simulink model "Ejercicio_1_DB_Inicial"  (R2023a)
settings: Solver=VariableStepAuto  StartTime=0.0  StopTime=150  RelTol=1e-6
values from neighbouring files (symbols this model uses):
  A = 10    [Ejercicio_1.m]    (also in Ejercicio_2y3.m)
  A1 = 1e-2    (= 0.01)    [Ejercicio_1.m]    (also in Ejercicio_2y3.m)
  A2 = 1    [Ejercicio_1.m]    (also in Ejercicio_2y3.m)
  bT = bm + (R*A1)^2*Rh + (R*A1/A2)^2*bp    (= 6.227045)    [Ejercicio_1.m]    (also in Ejercicio_2y3.m)
  JT = Jm + Jr + R^2*mp + (R*A1/A2)^2*m    (= 4.5108)    [Ejercicio_1.m]    (also in Ejercicio_2y3.m)
  Kb = 1    [Ejercicio_1.m]    (also in Ejercicio_2y3.m)
  kP = 5    [Ejercicio_1.m]    (also in Ejercicio_2y3.m)
  Kt = 1    [Ejercicio_1.m]    (also in Ejercicio_2y3.m)
  kT = (R*A1)^2/Ch + (R*A1/A2)^2*km    (= 0.26829)    [Ejercicio_1.m]    (also in Ejercicio_2y3.m)
  La = 100e-3    (= 0.1)    [Ejercicio_1.m]    (also in Ejercicio_2y3.m)
  R = 0.3    [Ejercicio_1.m]    (also in Ejercicio_2y3.m)
  Ra = 2.1    [Ejercicio_1.m]    (also in Ejercicio_2y3.m)
settings Model: Creator=54115  LastModifiedBy=franc
settings SolverCC: AlgebraicLoopSolver=TrustRegion
settings DebuggingCC: UnconnectedInputMsg=warning  UnconnectedOutputMsg=warning  UnconnectedLineMsg=warning
settings ModelReferenceCC: EnableRefExpFcnMdlSchedulingChecks=on

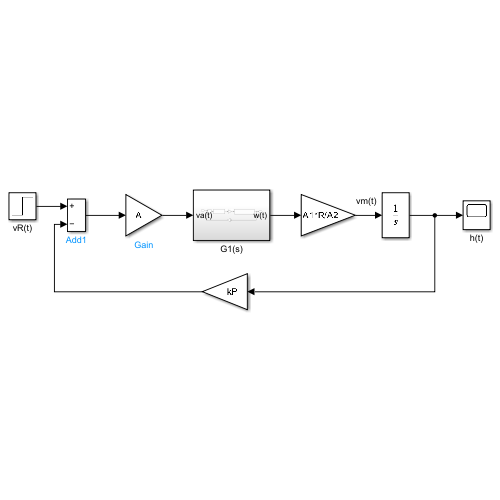
[thumbnail: Simulink's stored preview of the top-level diagram]
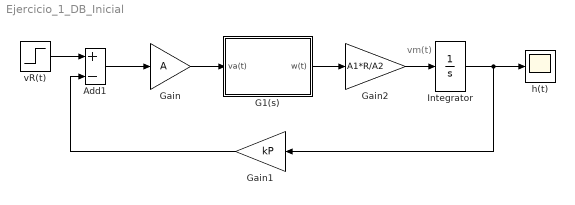
== system Ejercicio_1_DB_Inicial ==
  note: vm(t)
  Add1 : Sum  Inputs=+-
  G1(s) : Subsystem
  Gain : Gain  Gain=A
  Gain1 : Gain  Gain=kP
  Gain2 : Gain  Gain=A1*R/A2
  Integrator : Integrator
  h(t) : Scope
  vR(t) : Step  Time=0  SampleTime=0
  wires:
  vR(t)/1 -> Add1/1
  Gain1/1 -> Add1/2
  Add1/1 -> Gain/1
  Gain/1 -> G1(s)/1(va(t))
  G1(s)/1(w(t)) -> Gain2/1
  Gain2/1 -> Integrator/1
  Integrator/1 -> h(t)/1, Gain1/1

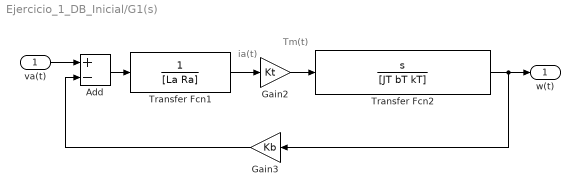
== system Ejercicio_1_DB_Inicial/G1(s) ==
  note: ia(t)
  note: Tm(t)
  va(t) : Inport
  Add : Sum  Inputs=+-
  Gain2 : Gain  Gain=Kt
  Gain3 : Gain  Gain=Kb
  Transfer Fcn1 : TransferFcn  Denominator=[La Ra]
  Transfer Fcn2 : TransferFcn  Numerator=[1 0]  Denominator=[JT bT kT]
  w(t) : Outport
  wires:
  Gain2/1 -> Transfer Fcn2/1
  Add/1 -> Transfer Fcn1/1
  Gain3/1 -> Add/2
  va(t)/1 -> Add/1
  Transfer Fcn2/1 -> w(t)/1, Gain3/1
  Transfer Fcn1/1 -> Gain2/1
